simulink model "h2t_TestBed_org"  (Simulink 10.0)
settings: Solver=FixedStepDiscrete  StartTime=0.0  StopTime=1  FixedStep=1  RelTol=1e-3  EnableMultiTasking=on
undefined symbols (not defined in the file): MWS
libraries: Lib_Thermo_Enth2Temp_TMATS x1
settings Model: Creator=jwchapm2  LastModifiedBy=annonymous
settings DataIOCC: LimitDataPoints=on
settings OptimizationCC: ExpressionDepthLimit=2147483647
settings DebuggingCC: SolverPrmCheckMsg=warning  StateNameClashWarn=warning
settings GRTTargetCC: GeneratePreprocessorConditionals=Disable all  CombineOutputUpdateFcns=on  GRTInterface=off
settings ConfigComp: CovExternalEMLEnable=off

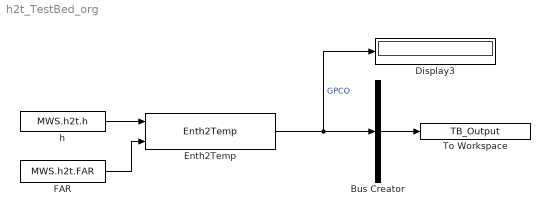
== system h2t_TestBed_org ==
  Bus Creator : BusCreator  Inputs=1
  Display3 : Display
  Enth2Temp : Lib_Thermo_Enth2Temp_TMATS/Enth2Temp
  FAR : Constant  Value=MWS.h2t.FAR
  To Workspace : ToWorkspace  VariableName=TB_Output  SampleTime=-1
  h : Constant  Value=MWS.h2t.h
  wires:
  FAR/1 -> Enth2Temp/2
  h/1 -> Enth2Temp/1
  Enth2Temp/1 -> Display3/1, Bus Creator/1  "GPCO"
  Bus Creator/1 -> To Workspace/1
